simulink model "vvvf"  (R2016a)
settings: Solver=ode23tb  SolverMode=SingleTasking  StartTime=0.0  StopTime=6  MaxStep=1e-4  RelTol=1e-3
undefined symbols (not defined in the file): magnitude
libraries: powerlib x5, powerlib_extras x2
settings Model: Creator=马鹏程  LastModifiedBy=马鹏程
settings DebuggingCC: SFUnexpectedBacktrackingDiag=error  SFNoUnconditionalDefaultTransitionDiag=error
settings GRTTargetCC: TargetLangStandard=C99 (ISO)
settings ConfigComp: CovMetricSettings=dwe  CovSaveCumulativeToWorkspaceVar=off  CovSaveSingleToWorkspaceVar=off  CovExternalEMLEnable=on

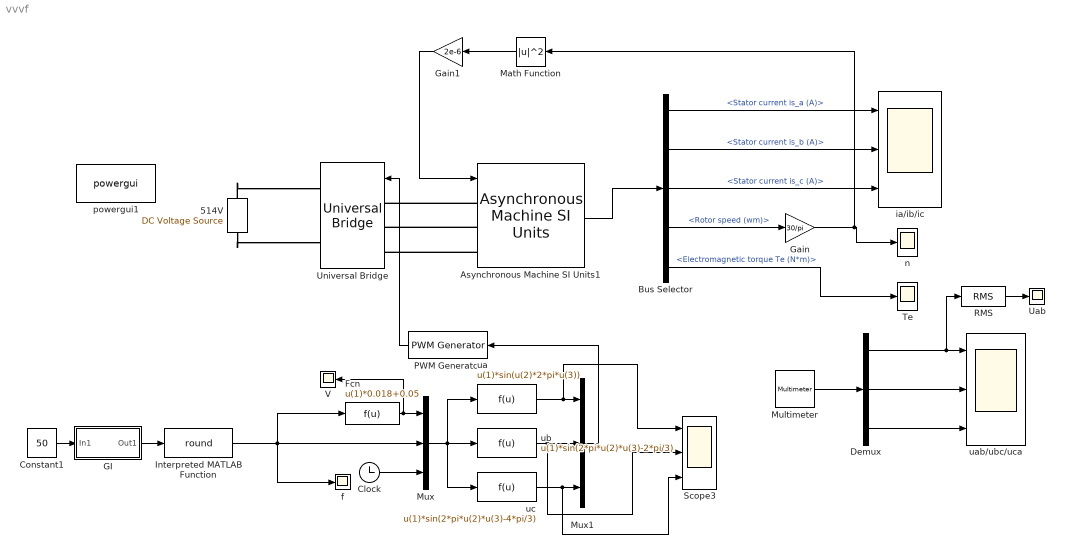
== system vvvf ==
  514V : powerlib/Electrical Sources/DC Voltage Source  Amplitude=514  Measurements=None
  Asynchronous Machine SI Units1 : powerlib/Machines/Asynchronous Machine SI Units  RotorType=Squirrel-cage  PresetModel="15:  5.4 HP (4KW)   400 V  50Hz 1430 RPM"  MechanicalLoad=Torque Tm  ShowDetailedParameters=on  ReferenceFrame=Rotor  Units=SI  MeasurementBus=off  NominalParameters=[4000 400 50]  Stator=[1.405 0.005839]  Rotor=[1.395 0.005839]  Cage1=[0.4155 0.002066]  Cage2=[0.4168 0.0003495]  Lm=0.1722  Mechanical=[0.0131 0.002985 2]  PolePairs=2  InitialConditions=[1 0 0 0 0 0 0 0]  SimulateSaturation=off  Saturation=[14.03593122, 27.81365428, 53.79336849, 72.68890987, 97.98006896, 148.6815601, 215.7428561, 302.9841135, 428.7778367 ; 230, 322, 414, 460, 506, 552, 598, 644, 690]  LoadFlowParameters=1492000  TsPowergui=0  TsBlock=-1  IterativeModel=Trapezoidal non iterative  IterativeDiscreteModel=Trapezoidal non iterative  Pmec=1.492e+006
  Bus Selector : BusSelector  OutputSignals=Stator measurements.Stator current is_a (A),Stator measurements.Stator current is_b (A),Stator measurements.Stator current is_c (A),Mechanical.Rotor speed (wm),Mechanical.Electromagnetic torque Te (N*m)
  Clock : Clock
  Constant1 : Constant  Value=50
  Demux : Demux  Outputs=3
  Fcn : Fcn  Expr=u(1)*0.018+0.05
  GI : Subsystem
  Gain : Gain  Gain=30/pi
  Gain1 : Gain  Gain=2e-6
  Interpreted MATLAB Function : MATLABFcn  MATLABFcn=round
  Math Function : Math  Operator=magnitude^2  SaturateOnIntegerOverflow=on
  Multimeter : powerlib/Measurements/Multimeter  PhasorSimulation=off  OutputType=Complex  sel=[1 2 3]  L=4  Gain=[1 1 1]  yselected={'Uab: Universal Bridge','Ubc: Universal Bridge','Uca: Universal Bridge'};  PSBOutputType=1  PSBequivalent=0  AxesSetting=[0,0.1,-100,100]  Display=0  SavedBlockNames=-11
  Mux : Mux  Inputs=3
  Mux1 : Mux  Inputs=3
  PWM Generator : powerlib_extras/Control  Blocks/PWM Generator  GeneratorMode="3-arm  bridge (6 pulses)"  Fc=1500  Internal=off  mIndex=0.4  Freq=60  Phase=0
  RMS : powerlib_extras/Measurements/RMS  f1=60
  Scope3 : Scope  NumInputPorts=3
  Te : Scope
  Uab : Scope
  Universal Bridge : powerlib/Power Electronics/Universal Bridge  Arms=3  SnubberResistance=1e5  SnubberCapacitance=inf  Device=IGBT / Diodes  Ron=1e-3  Lon=0  ForwardVoltages="[  1e-6, 2e-6 ]"  ForwardVoltage=0  GTOparameters=[ 10e-6 , 20e-6 ]  IGBTparameters=[ 1e-6 , 2e-6 ]  Measurements=UAB UBC UCA UDC voltages  Measurements_2=None  converterType=Rectifier
  V : Scope
  f : Scope
  ia/ib/ic : Scope  NumInputPorts=3
  n : Scope
  powergui1 : powerlib/powergui  Priority=1  SimulationMode=Continuous  SampleTime=50e-6  frequency=60  Iterations=50  frequencyindice=50  Pbase=100e6  ErrMax=1e-4  UnitsV=kV  UnitsW=MW  buscounter=0  FunctionMessages=off  echomessages=off  EnableUseOfTLC=off  CurrentSourceSwitches=off  DisableSnubberDevices=off  DisableRonSwitches=off  DisableVfSwitches=off  DisplayEquations=off  AutomaticDiscreteSolvers=off  SolverType=Tustin/Backward Euler (TBE)  Interpol=off  ExternalGateDelay=off  methode=off  Ts=100  x0status=blocks  SPID=on  SwTol=0  HookPort=off  NonlinearTolerance=1e-4  nMaxIteration=100  ContinueOnMaxIteration=off  RestoreLinks=warning  ResistiveCurrentMeasurement=off  Frange=[0:2:500]  Ylog=off  Xlog=on  ShowGrid=off  save=off  variable=ZData  structure=0  ZoomFFT=off  StartTime=0.0  cycles=1  DisplayStyle=1  fundamental=60  FreqAxis=off  MaxFrequency=1000  frequencyindicesteady=1  RmsSteady=1  display=off
  ua : Fcn  Expr=u(1)*sin(u(2)*2*pi*u(3))
  uab/ubc/uca : Scope  NumInputPorts=3
  ub : Fcn  Expr=u(1)*sin(2*pi*u(2)*u(3)-2*pi/3)
  uc : Fcn  Expr=u(1)*sin(2*pi*u(2)*u(3)-4*pi/3)
  wires:
  Asynchronous Machine SI Units1/1 -> Bus Selector/1
  Bus Selector/1 -> ia/ib/ic/1  "<Stator current is_a (A)>"
  Bus Selector/2 -> ia/ib/ic/2  "<Stator current is_b (A)>"
  Bus Selector/3 -> ia/ib/ic/3  "<Stator current is_c (A)>"
  Bus Selector/4 -> Gain/1  "<Rotor speed (wm)>"
  Gain/1 -> Math Function/1, n/1
  Bus Selector/5 -> Te/1  "<Electromagnetic torque Te (N*m)>"
  Mux1/1 -> PWM Generator/1
  Clock/1 -> Mux/3
  Mux/1 -> ub/1, ua/1, uc/1
  uc/1 -> Scope3/3, Mux1/3
  ua/1 -> Scope3/1, Mux1/1
  ub/1 -> Scope3/2, Mux1/2
  Constant1/1 -> GI/1(In1)
  Fcn/1 -> Mux/1, V/1
  PWM Generator/1 -> Universal Bridge/1
  Multimeter/1 -> Demux/1
  Demux/2 -> uab/ubc/uca/2
  Demux/3 -> uab/ubc/uca/3
  GI/1(Out1) -> Interpreted MATLAB Function/1
  Interpreted MATLAB Function/1 -> Mux/2, Fcn/1, f/1
  RMS/1 -> Uab/1
  Demux/1 -> RMS/1, uab/ubc/uca/1
  Math Function/1 -> Gain1/1
  Gain1/1 -> Asynchronous Machine SI Units1/1
  connections:
  Asynchronous Machine SI Units1/LConn1 -- Universal Bridge/LConn1
  Asynchronous Machine SI Units1/LConn2 -- Universal Bridge/LConn2
  Asynchronous Machine SI Units1/LConn3 -- Universal Bridge/LConn3
  514V/RConn1 -- Universal Bridge/RConn1
  514V/LConn1 -- Universal Bridge/RConn2

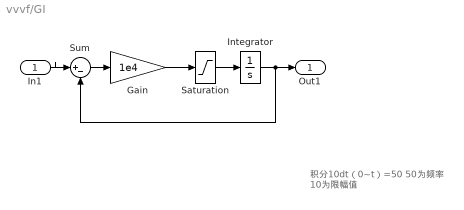
== system vvvf/GI ==
  note: 积分10dt（0~t）=50
      | 50为频率
      | 10为限幅值
  In1 : Inport
  Gain : Gain  Gain=1e4  SaturateOnIntegerOverflow=on  OutDataTypeStr=Inherit: Same as input  ParamDataTypeStr=Inherit: Same as input
  Integrator : Integrator
  Saturation : Saturate  UpperLimit=10  LowerLimit=-10
  Sum : Sum  Inputs=|+-  InputSameDT=on  SaturateOnIntegerOverflow=on  OutDataTypeStr=Inherit: Same as first input
  Out1 : Outport
  wires:
  Saturation/1 -> Integrator/1
  Gain/1 -> Saturation/1
  In1/1 -> Sum/1
  Integrator/1 -> Out1/1, Sum/2
  Sum/1 -> Gain/1
